simulink model "simul1"  (R2022a)
settings: Solver=VariableStepAuto  StartTime=0.0  StopTime=10.0  RelTol=1e-3
settings Model: Creator=radek  LastModifiedBy=radek
settings DebuggingCC: UnconnectedInputMsg=warning  UnconnectedOutputMsg=warning  UnconnectedLineMsg=warning
settings RTWCC: DLArmComputeVersion=19.05

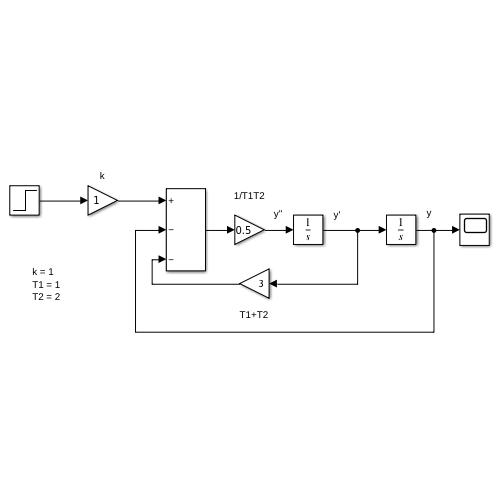
[thumbnail: Simulink's stored preview of the top-level diagram]
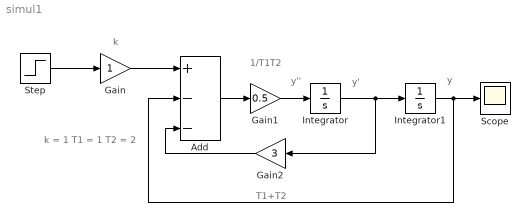
== system simul1 ==
  note: y
  note: y'
  note: y''
  note: T1+T2
  note: 1/T1T2
  note: k
  note: k = 1
      | T1 = 1
      | T2 = 2
  Add : Sum  Inputs=+--
  Gain : Gain
  Gain1 : Gain  Gain=0.5
  Gain2 : Gain  Gain=3
  Integrator : Integrator
  Integrator1 : Integrator
  Scope : Scope
  Step : Step  SampleTime=0
  wires:
  Add/1 -> Gain1/1
  Gain1/1 -> Integrator/1
  Integrator/1 -> Integrator1/1, Gain2/1
  Gain2/1 -> Add/3
  Integrator1/1 -> Add/2, Scope/1
  Gain/1 -> Add/1
  Step/1 -> Gain/1
